simulink model "PlanarChassisVehicleModel"  (R2021a)
settings: Solver=VariableStepAuto  StartTime=0.0  StopTime=10.0  RelTol=1e-3
(part 2 of 2)

== matlab function PlanarChassisVehicleModel/MATLAB Function13 ==
  data: Name input; Tire output; Source input; Notes input
function Tire = TireParameters(Name, Source, Notes)
%% TireParameters - Tire Model Structure Initialization
% This script generates an FRUCD tire model structure
% 
% Inputs:
%   Name   - (n,1 char)   Model Name
%   Source - (6,1 struct) Model Source File Information
%   Notes  - (n,1 cell)   Additional Model Notes
%
% Outputs:
%   Tire   - (1,1 struct) Initialized FRUCD Tire Model 
%
% Author(s): 
% Blake Christierson (bechristierson@ucdavis.edu) [Sep 2018 - Jun 2021] 
% 
% Last Updated: 02-May-2021

if nargin > 0
    Tire.Name    = Name;                      % Tire Name
    Tire.Date    = datestr(now,'dd-mm-yyyy'); % Generation Date
    Tire.Time    = datestr(now,'HH:MM PM'  ); % Generation Time
    Tire.Source  = Source;                    % Data Sources     
    Tire.Notes   = Notes;                     % Notes About Model

    Tire.Pacejka = PacejkaParameters();       % Pacejka Parameters
    Tire.Radius  = RadiusParameters();        % Radius Parameters
    Tire.Mass    = MassParameters();          % Mass Parameters
    Tire.Thermal = ThermalParameters();       % Thermal Parameters
end

function Pacejka = PacejkaParameters()
    %%% Nominal Conditions
    Pacejka.Fzo = 3000;       % Nominal Pacejka Load     [N] 
    Pacejka.Pio = 70;         % Nominal Pacejka Pressure [kPa]
    Pacejka.Ro  = 8*2.54/100; % Nominal Pacejka Radius   [m]
    Pacejka.Vo  = 15;         % Nominal Pacejka Velocity [m/s]
    
    % Scaling Factors (Lambdas)
    Pacejka.L.F.zo = 1; 

    Pacejka.L.mu.x = 1;
    Pacejka.L.mu.y = 1;
    Pacejka.L.mu.V = 0;

    Pacejka.L.K.x.k = 1;
    Pacejka.L.K.x.a = 1;

    Pacejka.L.K.y.a = 1;
    Pacejka.L.K.y.k = 1;

    Pacejka.L.K.y.g = 1;
    Pacejka.L.K.z.g = 1;

    Pacejka.L.C.x = 1;
    Pacejka.L.C.y = 1;
    Pacejka.L.C.z = 1;

    Pacejka.L.E.x = 1;
    Pacejka.L.E.y = 1;

    Pacejka.L.H.x = 1;
    Pacejka.L.H.y = 1;

    Pacejka.L.V.x = 1;
    Pacejka.L.V.y = 1;
    Pacejka.L.V.yk = 1;

    Pacejka.L.t = 1;

    Pacejka.L.M.x = 1;
    Pacejka.L.M.y = 1;
    Pacejka.L.M.r = 1;

    % Pacejka Spin Factors (Zetas)
    Pacejka.Z = ones(8,1);

    % p-Factors (Pure Slip Force Coefficients)
    Pacejka.p.C.x = 0;
    Pacejka.p.D.x = zeros(3,1);
    Pacejka.p.E.x = zeros(4,1);
    Pacejka.p.K.x = zeros(3,1);
    Pacejka.p.H.x = zeros(2,1);
    Pacejka.p.V.x = zeros(2,1);
    Pacejka.p.P.x = zeros(4,1);

    Pacejka.p.C.y = 0;
    Pacejka.p.D.y = zeros(3,1);
    Pacejka.p.E.y = zeros(5,1);
    Pacejka.p.K.y = zeros(7,1);
    Pacejka.p.H.y = zeros(2,1);
    Pacejka.p.V.y = zeros(4,1);
    Pacejka.p.P.y = zeros(5,1);

    % q-Factors (Moment Coefficients)
    Pacejka.q.B.z = zeros(10,1);
    Pacejka.q.C.z = 0;
    Pacejka.q.D.z = zeros(11,1);
    Pacejka.q.E.z = zeros(5,1);
    Pacejka.q.H.z = zeros(4,1);
    Pacejka.p.P.z = zeros(2,1);

    Pacejka.q.s.x = zeros(11,1);
    Pacejka.q.s.y = zeros(8,1);
    Pacejka.p.P.Mx = 0;
    
    % r-Factors (Combined Slip Force Coefficients)
    Pacejka.r.B.x = zeros(3,1);
    Pacejka.r.C.x = 0;
    Pacejka.r.E.x = zeros(2,1);
    Pacejka.r.H.x = 0;

    Pacejka.r.B.y = zeros(4,1);
    Pacejka.r.C.y = 0;
    Pacejka.r.E.y = zeros(2,1);
    Pacejka.r.H.y = zeros(2,1);
    Pacejka.r.V.y = zeros(6,1);

    % s-Factors (Combined Slip Aligning Moment Coefficients)
    Pacejka.s.s.z = zeros(4,1);
end

function Radius = RadiusParameters()
    Radius.Effective = [];
    Radius.Loaded    = [];
end

function Mass = MassParameters()
    Mass.m  = 0;            % Wheel Package Mass [kg]
    Mass.I  = zeros(3,3);   % Wheel Pacakge Inertia Tensor [kg-m^2]

    Mass.Is = 0;            % Spin Inertia (Spindle, Rotor, Rim, ...) [kg-m^2]
end

function Thermal = ThermalParameters()
    Thermal = [];
end

end

== matlab function PlanarChassisVehicleModel/MATLAB Function14 ==
  data: u input; y output
function y = fcn(u)

y = u;

== matlab function PlanarChassisVehicleModel/MATLAB Function1 ==
  data: LongVel input; Drag output; AirDensity input; RefArea input; DragCoeff input; LiftCoeff input; Downforce output
function [Drag, Downforce] = SimplifiedAeroLoads( LongVel, ...
    AirDensity, RefArea, DragCoeff, LiftCoeff )
%% SimplifiedWeightTransfer - Simplified Normal Loads
% Computes tire normal loads using simplified weight transfer and
% aerodynamic loading.
% 
% Inputs:
%   LongVel    - (n,1 numeric) Longitudinal Velocity {dot{x}}  [m/s]
%   AirDensity - (n,1 numeric) Air Density           {rho_air} [kg/m^3]
%   RefArea    - (n,1 numeric) Reference Area        {A}       [m^2]
%   DragCoeff  - (n,1 numeric) Drag Coefficient      {C_D}     [ ]
%   LiftCoeff  - (n,1 numeric) Lift Coefficient      {C_L}     [ ]
%
% Outputs:
%   Drag       - (n,1 numeric) Drag Force            {A_F_x}   [N]
%   Downforce  - (n,1 numeric) Downforce             {A_F_z}   [N]
%
% Notes:
%
% Author(s): 
% Blake Christierson (bechristierson@ucdavis.edu) [Sep 2018 - Jun 2021] 
% 
% Last Updated: 31-May-2021

%% Test Case
if nargin == 0
   LongVel = 15;
   
   AirDensity = 1.225;
   
   RefArea = 1.1;
   
   DragCoeff = 0.6;
   LiftCoeff = -1.9;
   
   [Drag, Downforce] = SimplifiedAeroLoads( LongVel, ...
    AirDensity, RefArea, DragCoeff, LiftCoeff ) %#ok<NOPRT>

    return
end

%% Computation
Drag      = 1/2 .* AirDensity .*  DragCoeff .* RefArea .* LongVel.^2;
Downforce = 1/2 .* AirDensity .* -LiftCoeff .* RefArea .* LongVel.^2;

end

== matlab function PlanarChassisVehicleModel/MATLAB Function ==
  data: PedalForce input; BrakingTorque output; PedalRatio input; BalanceBar input; BoreDiameter input; PadArea input; PadFriction input; RotorRadius input; LinePressure output
function [BrakingTorque, LinePressure] = SimplifiedBrakingModel( PedalForce, ...
    PedalRatio, BalanceBar  , BoreDiameter, ...
    PadArea   , PadFriction , RotorRadius )
%% SimplifiedBrakingModel - Braking Pressures and Torques
% Computes brake line pressure and braking torques assuming rigid braking
% components.
% 
% Inputs:
%   PedalForce   - (n,1 numeric) Pedal Force                   {F_p}   [N]
%   PedalRatio   - (n,1 numeric) Pedal Ratio                   {eta_p} [ ]
%   BalanceBar   - (n,1 numeric) Front Balance Bar Ratio       {%_bb}  [ ]
%   BoreDiameter - (n,2 numeric) Master Cylinder Bore Diameter {D_c}   [m]
%   PadArea      - (n,2 numeric) Brake Pad Area                {A_p}   [m^2]
%   PadFriction  - (n,2 numeric) Brake Pad Friction            {mu_p}  [ ]
%   RotorRadius  - (n,2 numeric) Brake Rotor Radius            {r_r}   [m]
%
% Outputs:
%   BrakingTorque - (n,4 numeric) Braking Torque      {tau_b} [N-m]
%   LinePressure  - (n,2 numeric) Brake Line Pressure {P_b}   [Pa]
%
% Notes:
%
% Author(s): 
% Blake Christierson (bechristierson@ucdavis.edu) [Sep 2018 - Jun 2021] 
% 
% Last Updated: 30-May-2021

%% Test Case
if nargin == 0
    PedalForce = 150;
    
    PedalRatio = 4.3;
    BalanceBar = 0.48;
    
    BoreDiameter = [0.59, 0.8125] .* 0.0254;
    
    PadArea = [2.9, 1.45] * 0.0254^2;
    PadFriction = [0.55, 0.55];
    
    RotorRadius = [3.3, 3.3] *0.0254;
    
    [BrakingTorque, LinePressure] = SimplifiedBrakingModel( PedalForce, ...
        PedalRatio, BalanceBar  , BoreDiameter, ...
        PadArea   , PadFriction , RotorRadius ) %#ok<NOPRT>
    
    return
end

%% Computation
CylinderForce = PedalForce .* PedalRatio .* [BalanceBar, 1-BalanceBar];

LinePressure = CylinderForce ./ (pi/4 .* BoreDiameter.^2);

BrakingTorque = LinePressure .* PadArea .* PadFriction .* LinePressure / 2;
BrakingTorque = [BrakingTorque(:,1).*ones(1,2), BrakingTorque(:,2).*ones(1,2)];

end

== matlab function PlanarChassisVehicleModel/MATLAB Function3 ==
  data: Yaw input; GlobLongVel output; LatAcc input; LatVel input; LongAcc input; LongVel input; GlobLatVel output; Curvature output; BodySlipAngle output
function [GlobLongVel, GlobLatVel, Curvature, BodySlipAngle] = ...
    BicycleModelWCS( Yaw, LatAcc, LatVel, LongAcc, LongVel )

%% WCS - World Coordinate System Calculations
% 
% Inputs:
%  Yaw     - (n,1 numeric) Yaw                       {psi} [rad]
%  LatAcc  - (n,1 numeric) Lateral Acceleration      {y_ddot} [m/s^2]
%  LatVel  - (n,1 numeric) Lateral Velocity          {y_dot} [m/s]
%  LongAcc - (n,1 numeric) Longitudinal Acceleration {x_ddot} [m/s^2]
%  LongVel - (n,1 numeric) Longitudinal Velocity     {x_dot} [m/s]
% 
% Outputs:
%  GlobLongVel   - (n,1 numeric) Global Longitudial Velocity {X_dot} [m/s]
%  GlobLatVel    - (n,1 numeric) Golbal Lateral Velocity     {Y_dot} [m/s]
%  Curvature     - (n,1 numeric) Pedal Force                 {R} [m]
%  BodySlipAngle - (n,1 numeric) Body Slip Angle             {beta} [degrees]
%  
% Notes:
% Naming convention for R still not in place
%
% Author(s): 
% Tristan Pham (atlpham@ucdavis.edu) [Sep 2020 - Jun 2021] 

% Last Updated: 27-Mar-2021


%% Test Cases
if nargin == 0
    %%% Test Inputs
    Yaw = ; 
    
    LatAcc = ; 
    LatVel = ; 
    
    LongAcc = ;
    LongVel = ;
    
  
    
    fprintf('Executing World Coordinate System() Test Cases: \n');
    
    
    [GlobLongVel, GlobLatVel, Curvature, BodySlipAngle] = BicycleModelWCS( Yaw, ...
        LatAcc, LatVel, LongAcc, LongVel);
    
 % for i = 1:numel()
      %  fprintf('   Steady State Instance %i: \n', i);
      % fprintf('      tau_i = %5.2f [N-m] \n', InputTorque(i));
   % end
    
    
     %return;   
end
    
%% Computation

% Global Velocity
GlobLongVel = LongVel .* cosd( Yaw ) - LatVel .* sind( Yaw );
GlobLatVel = LongVel .* sind( Yaw ) + LatVel .* cosd( Yaw );  
                 
% Curvature
if abs(LongVel.^2 + LatVel.^2) <= 0.01
    Curvature = 0;
else
    Curvature = ( LatVel.^2 + LatVel.^2 ).^(3/2) ./ ...
        abs( LongAcc.*LatVel - LongVel.*LatAcc );
end

% Body Slip
BodySlipAngle = atan2d( LatVel, LongVel );

== matlab function PlanarChassisVehicleModel/MATLAB Function4 ==
  data: TFx input; LongAcc output; TFy input; TMz input; AFx input; AFy input; AMz input; Wheelbase input; TrackWidth input; Steer input; Mass input; YawInertia input; CoG input; LongVel input; LatVel input; YawVel input; LatAcc output; YawAcc output; LongAccTot output; LatAccTot output
function [LongAcc, LatAcc, YawAcc, LongAccTot, LatAccTot] = ...
    FullTrack3DOFAccelerations( TFx, TFy, TMz, AFx, AFy, AMz, ... % Loads
        Wheelbase, TrackWidth, Steer, ...                         % Geometry
        Mass, YawInertia, CoG, ...                                % Inertia
        LongVel, LatVel, YawVel )                                 % Velocities
%% FullTrack3DOFAccelerations - Full Track Planar Accelerations
% Computes planar motion accelerations for a 3DOF full track chassis model
% 
% Inputs:
%   TFx        - (n,4 numeric) Tire Longitudinal Force {T_F_y}    [N]
%   TFy        - (n,4 numeric) Tire Lateral Force      {T_F_y}    [N]
%   TMz        - (n,4 numeric) Tire Aligning Moment    {T_M_z}    [N-m]
%   AFx        - (n,1 numeric) Aerodynamic Drag Force  {A_F_x}    [N]
%   AFy        - (n,1 numeric) Aerodynamic Side Force  {A_F_y}    [N]
%   AMz        - (n,1 numeric) Aerodynamic Yaw Moment  {A_M_z}    [N-m]
%   Wheelbase  - (n,1 numeric) Wheelbase               {L}        [m]
%   TrackWidth - (n,2 numeric) Track Width             {t_w}      [m]
%   Steer      - (n,4 numeric) Tire Steer Angle        {delta}    [deg]
%   Mass       - (n,1 numeric) Total Vehicle Mass      {m}        [kg]
%   YawInertia - (n,1 numeric) Vehicle Yaw Inertia     {I_zz}     [kg-m^2]
%   CoG        - (n,3 numeric) Center of Gravity       {CoG}      [m]
%   LongVel    - (n,1 numeric) Longitudinal Velocity   {dot{x}}   [m/s]
%   LatVel     - (n,1 numeric) Lateral Velocity        {dot{y}}   [m/s]
%   YawVel     - (n,1 numeric) Yaw Velocity            {dot{psi}} [rad/s]
%
% Outputs:
%   LongAcc    - (n,1 numeric) Longitudinal Acceleration       {ddot{x}}  [m/s^2]
%   LatAcc     - (n,1 numeric) Lateral Acceleration            {ddot{y}}  [m/s^2]
%   YawAcc     - (n,1 numeric) Yaw Acceleration                {ddot{psi} [rad/s^2]
%   LongAccTot - (n,1 numeric) Total Longitudinal Acceleration {a_x}      [m/s^2]
%   LatAccTot  - (n,1 numeric) Total Lateral Acceleration      {a_y}      [m/s^2]
%
% Notes:
%
% Author(s): 
% Blake Christierson (bechristierson@ucdavis.edu) [Sep 2018 - Jun 2021] 
% Tristan Pham       (atlpham@ucdavis.edu)        [Oct 2020 - ???     ]
% 
% Last Updated: 30-May-2021

%% Test Case
if nargin == 0
    TFx = zeros(1,4);
    TFy = [250, 250, 0, 0];
    TMz = zeros(1,4);
    
    AFx = -100;
    AFy = 0;
    AMz = 0;
    
    Wheelbase  = 1.575; 
    TrackWidth = 1.22*ones(1,2);
    Steer      = [18, 15, 1, -1];
    
    Mass       = 275;   
    YawInertia = 130; 
    CoG        = [(0.47-0.5)*Wheelbase, 0, 0.25];
    
    LongVel = 15;
    LatVel  = 0;
    YawVel  = 0.5;
    
    [LongAcc, LatAcc, YawAcc, LongAccTot, LatAccTot] = ...
        FullTrack3DOFAccelerations( ...
            TFx, TFy, TMz, AFx, AFy, AMz, ...
            Wheelbase, TrackWidth, Steer, ... 
            Mass, YawInertia, CoG, ... 
            LongVel, LatVel, YawVel ) %#ok<NOPRT>
    
    return;
end

%% Computations
%%% Tire Positions (n,4,3 numeric)
TirePos = cat( 3, Wheelbase/2 + [-1, -1, 1, 1].*CoG(:,1), ...
                  [TrackWidth(:,1).*[1 -1]/2, TrackWidth(:,2).*[1 -1]/2], ...
                  zeros( size(Steer) ) );

%%% Tire Loads (n,4,3 numeric)
TireLoad = cat( 3, TFx, TFy, zeros( size(Steer) ) );

%%% Tire Yaw Moment (n,1 numeric)
TireMoment = cross(TirePos, TireLoad, 3);
TireMoment = sum( TireMoment(:,:,3) ) + sum(TMz,2);

%%% Chassis Accelerations
LongAcc = (sum( TFx.*cosd(Steer) - TFy.*sind(Steer), 2 ) + LatVel.*YawVel  - AFx) ./ Mass;
LatAcc  = (sum( TFy.*cosd(Steer) + TFx.*sind(Steer), 2 ) - LongVel.*YawVel - AFy) ./ Mass;
YawAcc  = (TireMoment - AMz) ./ YawInertia;

LongAccTot = LongAcc - LatVel .*YawVel;
LatAccTot  = LatAcc  + LongVel.*YawVel;

== matlab function PlanarChassisVehicleModel/MATLAB Function5 ==
  data: SpinRate input; DriveTorque output; AxleTorque input; BrakePreload input; DrivePreload input; DeltaTorque output
function [DriveTorque, DeltaTorque] = DifferentialModel(SpinRate, AxleTorque, BrakePreload, DrivePreload )
%% DifferentialModel - Drive Torque and Delta Torque Calculations 
% Estimates the diffrential's drive torque and delta torque from the
% spin rate, axle torque, and a set of parameters. To avoid differential
% algebaric equations the relaxtion technique was applied to delta torque.
%
% Inputs:
%   AxleTorque          - (1,1 numeric) Axle Drive Torquw                   {tau_A}   [Nm]
%   SpinRate            - (n,1 numeric) Rear Wheel Spin Rate                {omega}   [rad/s]
%   BrakePreload        - (1,1 numeric) Brake Torque Preload                {tau_B}   [Nm]
%   DrivePreload        - (1,1 numeric) Drive Torque Preload                {tau_D}   [Nm]
%   RampRadius          - (1,1 numeric) Ramp Radius                         {r_o}     [m]
%   DriveRampAngle      - (1,1 numeric) Drive Ramp Angle                    {sigma_D} [deg]
%   BrakeRampAngle      - (1,1 numeric) Brake Ramp Angle                    {sigma_B} [deg]
%   ClutchOuterRadius   - (1,1 numeric) Clutch Pack Outer Radius            {r_o}     [m] 
%   ClutchInnerRadius   - (1,1 numeric) Clutch Pack Inner Radius            {r_i}     [m]
%   ClutchCoeffFriction - (1,1 numeric) Clutch Pack Coefficient of Friction {mu_c}    []
%   NumbFrictionSurface - (1,1 numeric) Number of Friction Surfaces         {N}       []
% State: 
%   DeltaSpinRate - (1,1 numeric) Delta of Rear SpinRates {Delta*omega} [rad/s]
%
% Output:
%   DriveTorque - (1,1 numeric) Drive Torque        {tau_D}     [Nm]
%   DeltaTorque - (n,1 numeric) Differential Torque {Delta*tau} [Nm]

%Note:
%delT = (Ta/rramp) *.cot(sigma_d)).*(2/3 * ((ro^3 - ri ^3) / (ro^2-ro^2))(mu_c *N)*(abs(DeltaOmega)*tanh(4abs(DeltaOmega)
%Is not implemented. 

%Author(s):
%Joseph Sanchez (jomsanchez@ucdavis.edu)

%Last Updates: 4-Apr-2021

%%% Test Case 

if nargin == 0 
    SpinRate     = 10*ones(1,4);
    AxleTorque   = 15;
    BrakePreload = 1;
    DrivePreload = 5; 

    [DriveTorque, DeltaTorque] = DifferentialModel(SpinRate, AxleTorque,...
        BrakePreload, DrivePreload );
    
        fprintf('Executing WheelSpeed() Test Case: \n');
        for i = 1:numel(DriveTorque)
            fprintf('   Instance %i: \n', i);
            fprintf('      DriveTorque = %5.2f [Nm] \n', DriveTorque(i));
            
        end 
        
            return;
end 
%% Differential Spin Rate
DeltaSpinRate = SpinRate(3) - SpinRate(4);

%% Differential Torque 
DriveTorque = zeros(1,4);

if (AxleTorque > BrakePreload) && (AxleTorque < DrivePreload) %Is Locked 
    DeltaTorque = ( AxleTorque*0.5)*(tanh(100*DeltaSpinRate)); %Insert delT here once obtained parameter values   
else 
    DeltaTorque = ( AxleTorque*0.5)*(tanh(4*DeltaSpinRate));   
end

DriveTorque(3) = 0.5*AxleTorque - sign(DeltaSpinRate)*DeltaTorque; 
DriveTorque(4) = 0.5*AxleTorque + sign(DeltaSpinRate)*DeltaTorque;


end
